simulink model "controllo_Completo_v14"  (R2025a)
settings: Solver=VariableStepAuto  StartTime=0.0  StopTime=Durata_Simulazione  MaxStep=Passo_integrazione_massimo  RelTol=1e-3
values from neighbouring files (symbols this model uses):
  C_bat_eq_rx = 1.0    (= 1)    [p_schema_completo_generale_v2.m]
  C_bat_eq_tx = 3.5    [p_schema_completo_generale_v2.m]
  C_bus_dc_dc = 1.5e-3    (= 0.0015)    [p_schema_completo_generale_v2.m]
  C_ris = 1/(w_dc_ac_nom^2*L_coil)    (= 6.49245057301e-08)    [p_schema_completo_generale_v2.m]
  dead_time_dc_dc = 0.3e-6    (= 3e-07)    [p_schema_completo_generale_v2.m]
  duty_A_0_tx = V_bat_0_tx/V_dc_0_tx    (= 0.472727272727)    [p_schema_completo_generale_v2.m]
  duty_B_0_tx = duty_A_0_tx    (= 0.472727272727)    [p_schema_completo_generale_v2.m]
  duty_leg_A_dc_dc_0_tx = V_bat_0_tx/V_dc_0_tx    (= 0.472727272727)    [p_schema_completo_generale_v2.m]
  duty_leg_B_dc_dc_0_tx = duty_leg_A_dc_dc_0_tx    (= 0.472727272727)    [p_schema_completo_generale_v2.m]
  Ibat_rif_max = 50    [p_schema_completo_generale_v2.m]
  Ibat_rif_min = -50    [p_schema_completo_generale_v2.m]
  Kp_P_tensione_batteria_rx = 1/modulo_catena_aperta_tensione_batteria_reg_P_rx    [p_schema_completo_generale_v2.m]
  Kp_P_tensione_batteria_tx = 1/modulo_catena_aperta_tensione_batteria_reg_P_tx    [p_schema_completo_generale_v2.m]
  L_coil = 54e-6    (= 5.4e-05)    [p_schema_completo_generale_v2.m]
  L_filtro_dc_dc = 65e-6    (= 6.5e-05)    [p_schema_completo_generale_v2.m]
  M_coil = k*sqrt(L_coil^2)    [p_schema_completo_generale_v2.m]
  Parametri_Controllori = [Parametri_Controllori     PI_corrente_trasm_tf_disc_den(2) PI_corrente_trasm_tf_disc_num(1) PI_corrente_trasm_tf_disc_num(2)]    [p_schema_completo_generale_v2.m]
  R_bat = 32e-3    (= 0.032)    [p_schema_completo_generale_v2.m]
  R_coil = w_dc_ac_nom*L_coil/Q_coil    (= 0.2883982056)    [p_schema_completo_generale_v2.m]
  R_coil_M = sqrt(w_dc_ac_nom^2)*M_coil/sqrt(Q_coil^2)    [p_schema_completo_generale_v2.m]
  R_Lfiltro_dc_dc = 6.5e-3    (= 0.0065)    [p_schema_completo_generale_v2.m]
  Req_Lfiltro_dc_dc = (R_Lfiltro_dc_dc+Rds_on_dc_dc)    (= 0.0075)    [p_schema_completo_generale_v2.m]
  Rshunt_coil = 1e5    (= 100000)    [p_schema_completo_generale_v2.m]
  Rshunt_Lfiltro = 1e6    (= 1000000)    [p_schema_completo_generale_v2.m]
  T_dc_ac = 1/freq_dc_ac    (= 1.17647058824e-05)    [p_schema_completo_generale_v2.m]
  T_dc_dc = 1/freq_dc_dc    (= 7.8431372549e-06)    [p_schema_completo_generale_v2.m]
  tau_filtro_anti_aliasing = R_filtro_anti_aliasing*C_filtro_anti_aliasing    (= 1.96e-06)    [p_schema_completo_generale_v2.m]
  tau_filtro_pb_coil = 1/(2*pi*f_filtro_pb_coil)    (= 3.18309886184e-05)    [p_schema_completo_generale_v2.m]
  tau_filtro_pb_corrente_bat = 1/(2*pi*f_filtro_pb_corrente_bat)    (= 2.49654812693e-05)    [p_schema_completo_generale_v2.m]
  Ts_BMS = 1e-3    (= 0.001)    [p_schema_completo_generale_v2.m]
  Ts_dc_ac = 4*T_dc_ac    (= 4.70588235294e-05)    [p_schema_completo_generale_v2.m]
  Ts_dc_dc = Ts_dc_ac    (= 4.70588235294e-05)    [p_schema_completo_generale_v2.m]
  Ts_trasmissione = 1e-3    (= 0.001)    [p_schema_completo_generale_v2.m]
  V_bat_0_rx = V_bat_nom    (= 96)    [p_schema_completo_generale_v2.m]
  V_bat_0_tx = V_bat_max-5    (= 104)    [p_schema_completo_generale_v2.m]
  V_bat_max = 109    [p_schema_completo_generale_v2.m]
  V_bat_max_alg = 218    [Controllo_tensione_bus_dc.m]    (also in Controllo_tensione_bus_dc_corrente_bobina.m; p_schema_completo_generale_v2.m)
  V_bat_min = 75    [p_schema_completo_generale_v2.m]
  V_bat_min_alg = 37.5    [Controllo_tensione_bus_dc.m]    (also in Controllo_tensione_bus_dc_corrente_bobina.m; p_schema_completo_generale_v2.m)
  V_dc_0_rx = 230    [p_schema_completo_generale_v2.m]
  V_dc_0_tx = 220    [p_schema_completo_generale_v2.m]
  Vbat_rif_max_tx = V_bat_max    (= 109)    [p_schema_completo_generale_v2.m]
  Vbat_rif_min_tx = V_bat_min    (= 75)    [p_schema_completo_generale_v2.m]
  Vdc_rif_max_tx = V_dc_nom+5    (= 255)    [p_schema_completo_generale_v2.m]
  Vdc_rif_min_tx = V_dc_nom-5    (= 245)    [p_schema_completo_generale_v2.m]
undefined symbols (not defined in the file or in its folder): Ceq_bat_tx, Cris_tx, Lfilt_dc_dc, Lfiltro_dc_dc_tx, R_bat_rx, R_bat_tx
libraries: simulink x44, spsSeriesRLCBranchLib x36, spsCurrentMeasurementLib x20, spsMosfetLib x16, spsVoltageMeasurementLib x12, simulink_extras x4, spsControlledCurrentSourceLib x4, spsControlledVoltageSourceLib x4, spsDCVoltageSourceLib x2, spsMutualInductanceLib x1, spsGroundLib x1, sps_lib x1
(part 3 of 7)

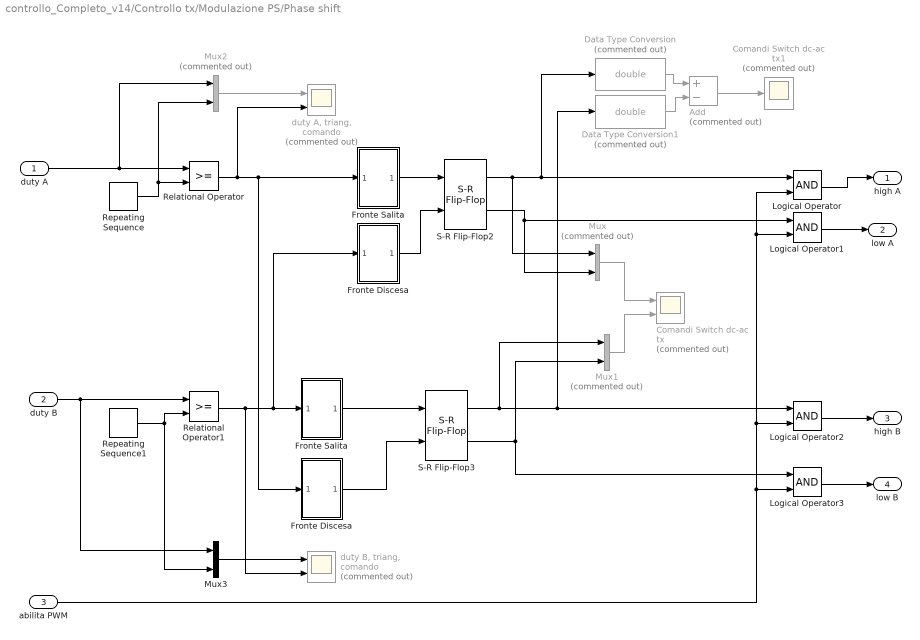
== system controllo_Completo_v14/Controllo tx/Modulazione PS/Phase shift ==
  duty A : Inport
  duty B : Inport  Port=2
  abilita PWM : Inport  Port=3
  Add : Sum  Commented=on  Inputs=+-
  Comandi Switch dc-ac tx : Scope  Commented=on  NumInputPorts=2
      settings: ActiveDisplayYMinimum=-0.12499999999999997  ActiveDisplayYMaximum=1.125  DataLoggingVariableName=ScopeData14
  Comandi Switch dc-ac tx1 : Scope  Commented=on
      settings: ActiveDisplayYMinimum=-1.25  ActiveDisplayYMaximum=1.25  DataLoggingVariableName=ScopeData5
  Data Type Conversion : DataTypeConversion  Commented=on  OutDataTypeStr=double  SaturateOnIntegerOverflow=off  RndMeth=Floor
  Data Type Conversion1 : DataTypeConversion  Commented=on  OutDataTypeStr=double  SaturateOnIntegerOverflow=off  RndMeth=Floor
  Fronte Discesa : Subsystem
  "Fronte Discesa " : Subsystem
  Fronte Salita : Subsystem
  "Fronte Salita " : Subsystem
  Logical Operator{,1..3} (4 alike) : Logic  AllPortsSameDT=off  OutDataTypeStr=boolean
  Mux : Mux  Commented=on  Inputs=2
  Mux1 : Mux  Commented=on  Inputs=2
  Mux2 : Mux  Commented=on  Inputs=2
  Mux3 : Mux  Inputs=2
  Relational Operator : RelationalOperator  OutDataTypeStr=boolean  RndMeth=Simplest  InputSameDT=off
  Relational Operator1 : RelationalOperator  OutDataTypeStr=boolean  RndMeth=Simplest  InputSameDT=off
  Repeating Sequence : simulink/Sources/Repeating Sequence  rep_seq_t=[0 1/2 1]*T_dc_ac  rep_seq_y=[1 0 1]
  Repeating Sequence1 : simulink/Sources/Repeating Sequence  rep_seq_t=[0 1/2 1]*T_dc_ac  rep_seq_y=[1 0 1]
  S-R Flip-Flop2 : simulink_extras/Flip Flops/S-R Flip-Flop  initial_condition=0
  S-R Flip-Flop3 : simulink_extras/Flip Flops/S-R Flip-Flop  initial_condition=0
  "duty A, triang, comando" : Scope  Commented=on  NumInputPorts=2
      settings: ActiveDisplayYMinimum=0.98956207928910589  ActiveDisplayYMaximum=1.00212977441315  DataLoggingVariableName=ScopeData29
  "duty B, triang, comando" : Scope  Commented=on  NumInputPorts=2
      settings: ActiveDisplayYMinimum=-0.12499999999999997  ActiveDisplayYMaximum=1.125  DataLoggingVariableName=ScopeData24
  high A : Outport
  low A : Outport  Port=2
  high B : Outport  Port=3
  low B : Outport  Port=4
  wires:
  Repeating Sequence/1 -> Mux2/2, Relational Operator/2
  duty B/1 -> Mux3/1, Relational Operator1/1
  Relational Operator/1 -> "duty A, triang, comando"/2, "Fronte Discesa "/1(In1), Fronte Salita/1(In1)
  Relational Operator1/1 -> "duty B, triang, comando"/2, "Fronte Salita "/1(In1), Fronte Discesa/1(In1)
  Repeating Sequence1/1 -> Mux3/2, Relational Operator1/2
  duty A/1 -> Mux2/1, Relational Operator/1
  Mux/1 -> Comandi Switch dc-ac tx/1
  Mux1/1 -> Comandi Switch dc-ac tx/2
  Fronte Salita/1(Out1) -> S-R Flip-Flop2/1
  Fronte Discesa/1(Out1) -> S-R Flip-Flop2/2
  S-R Flip-Flop2/1 -> Mux/1, Data Type Conversion/1, Logical Operator/1
  S-R Flip-Flop2/2 -> Mux/2, Logical Operator1/1
  "Fronte Salita "/1(Out1) -> S-R Flip-Flop3/1
  "Fronte Discesa "/1(Out1) -> S-R Flip-Flop3/2
  S-R Flip-Flop3/1 -> Mux1/1, Logical Operator2/1, Data Type Conversion1/1
  S-R Flip-Flop3/2 -> Mux1/2, Logical Operator3/1
  Add/1 -> Comandi Switch dc-ac tx1/1
  Data Type Conversion/1 -> Add/1
  Data Type Conversion1/1 -> Add/2
  Mux2/1 -> "duty A, triang, comando"/1
  Mux3/1 -> "duty B, triang, comando"/1
  Logical Operator/1 -> high A/1
  Logical Operator1/1 -> low A/1
  Logical Operator2/1 -> high B/1
  Logical Operator3/1 -> low B/1
  abilita PWM/1 -> Logical Operator3/2, Logical Operator2/2, Logical Operator1/2, Logical Operator/2

== system controllo_Completo_v14/Controllo tx/Modulazione PWM/Variant Subsystem ==
  high A : Inport
  low A : Inport  Port=2
  high B : Inport  Port=3
  low B : Inport  Port=4
  dead time : Subsystem  VariantControl=(Selettore_No_Dead_Time_0_Dead_Time_1_tx==1)&(Selettore_Switching_0_Valori_Medi_1_dc_dc_tx==0)
  no dead time : Subsystem  VariantControl=(Selettore_No_Dead_Time_0_Dead_Time_1_tx==0)|(Selettore_Switching_0_Valori_Medi_1_dc_dc_tx==1)
  high A DT : Outport
  low A DT : Outport  Port=2
  high B DT : Outport  Port=3
  low B DT : Outport  Port=4

== system controllo_Completo_v14/Controllo tx/Modulazione PWM/Variant Subsystem1 ==
  duty A : Inport
  duty B : Inport  Port=2
  abilita PWM : Inport  Port=3
  Modulazione Lineare : Subsystem  VariantControl=Selettore_Switching_0_Valori_Medi_1_dc_dc_tx==1
  PWM Seno-Triangolo : Subsystem  VariantControl=Selettore_Switching_0_Valori_Medi_1_dc_dc_tx==0
  high A : Outport
  low A : Outport  Port=2
  high B : Outport  Port=3
  low B : Outport  Port=4

== system controllo_Completo_v14/Convertitore dc-dc/Convertitore dc-dc valori medi/Subsystem ==
  From : From  Commented=on  GotoTag=dc_dc_leg_A_high_tx  TagVisibility=global
  From11 : From  Commented=on  GotoTag=v_dc_tx  TagVisibility=global
  From12 : From  Commented=on  GotoTag=v_bat_tx  TagVisibility=global
  From13 : From  Commented=on  GotoTag=v_dc_tx  TagVisibility=global
  From18 : From  Commented=on  GotoTag=v_bat_tx  TagVisibility=global
  From5 : From  Commented=on  GotoTag=dc_dc_leg_B_high_tx  TagVisibility=global
  From7 : From  Commented=on  GotoTag=abilita_PWM_tx  TagVisibility=global
  Product2 : Product  Commented=on
  Product4 : Product  Commented=on
  Switch : Switch  Commented=on  Criteria=u2 > Threshold  Threshold=0.5  SaturateOnIntegerOverflow=off  InputSameDT=off
  Switch1 : Switch  Commented=on  Criteria=u2 > Threshold  Threshold=0.5  SaturateOnIntegerOverflow=off  InputSameDT=off
  Out1 : Outport
  Out2 : Outport  Port=2
  wires:
  From7/1 -> Switch1/2, Switch/2
  From18/1 -> Switch1/3
  From5/1 -> Product4/2
  Product4/1 -> Switch1/1
  From11/1 -> Product2/1
  From12/1 -> Switch/3
  Product2/1 -> Switch/1
  Switch/1 -> Out1/1
  From/1 -> Product2/2
  From13/1 -> Product4/1
  Switch1/1 -> Out2/1

== system controllo_Completo_v14/Convertitore dc-dc /Convertitore dc-dc Valori Medi /Subsystem ==
  From13 : From  Commented=on  GotoTag=dc_dc_leg_A_high_rx  TagVisibility=global
  From14 : From  Commented=on  GotoTag=dc_dc_leg_B_high_rx  TagVisibility=global
  From20 : From  Commented=on  GotoTag=abilita_PWM_rx  TagVisibility=global
  From21 : From  Commented=on  GotoTag=v_dc_rx  TagVisibility=global
  From22 : From  Commented=on  GotoTag=v_bat_rx  TagVisibility=global
  From23 : From  Commented=on  GotoTag=v_dc_rx  TagVisibility=global
  Product3 : Product  Commented=on
  Product8 : Product  Commented=on
  Switch2 : Switch  Commented=on  Criteria=u2 > Threshold  Threshold=0.5  SaturateOnIntegerOverflow=off  InputSameDT=off
  Switch3 : Switch  Commented=on  Criteria=u2 > Threshold  Threshold=0.5  SaturateOnIntegerOverflow=off  InputSameDT=off
  Out1 : Outport
  Out2 : Outport  Port=2
  wires:
  Switch2/1 -> Out1/1
  From14/1 -> Product8/2
  From21/1 -> Product3/1
  Switch3/1 -> Out2/1
  From22/1 -> Switch3/3, Switch2/3
  Product8/1 -> Switch3/1
  Product3/1 -> Switch2/1
  From23/1 -> Product8/1
  From20/1 -> Switch3/2, Switch2/2
  From13/1 -> Product3/2

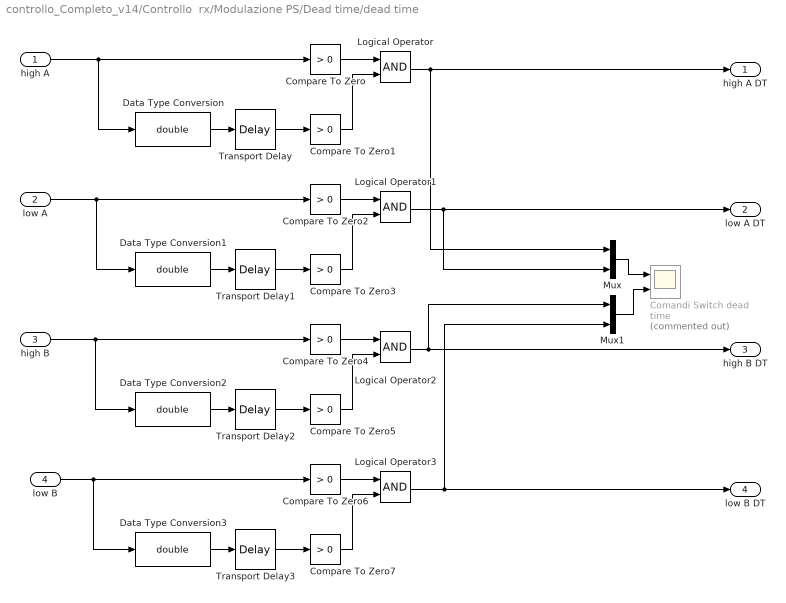
== system controllo_Completo_v14/Controllo  rx/Modulazione PS/Dead time/dead time ==
  high A : Inport
  low A : Inport  Port=2
  high B : Inport  Port=3
  low B : Inport  Port=4
  Comandi Switch dead time : Scope  Commented=on  NumInputPorts=2
      settings: ActiveDisplayYMinimum=-0.12499999999999997  ActiveDisplayYMaximum=1.125  DataLoggingVariableName=ScopeData11
  Compare To Zero{,1..7} (8 alike) : simulink/Logic and Bit Operations/Compare To Zero  relop=>  OutDataTypeStr=boolean
  Data Type Conversion{,1..3} (4 alike) : DataTypeConversion  OutDataTypeStr=double  SaturateOnIntegerOverflow=off  RndMeth=Floor
  Logical Operator{,1..3} (4 alike) : Logic  AllPortsSameDT=off  OutDataTypeStr=boolean
  Mux : Mux  Inputs=2
  Mux1 : Mux  Inputs=2
  Transport Delay{,1..3} (4 alike) : TransportDelay  DelayTime=dead_time_dc_dc
  high A DT : Outport
  low A DT : Outport  Port=2
  high B DT : Outport  Port=3
  low B DT : Outport  Port=4
  wires:
  Mux/1 -> Comandi Switch dead time/1
  Data Type Conversion3/1 -> Transport Delay3/1
  Data Type Conversion2/1 -> Transport Delay2/1
  Data Type Conversion1/1 -> Transport Delay1/1
  Data Type Conversion/1 -> Transport Delay/1
  Mux1/1 -> Comandi Switch dead time/2
  Logical Operator2/1 -> high B DT/1, Mux1/1
  Logical Operator3/1 -> low B DT/1, Mux1/2
  high B/1 -> Data Type Conversion2/1, Compare To Zero4/1
  Transport Delay2/1 -> Compare To Zero5/1
  Compare To Zero5/1 -> Logical Operator2/2
  Compare To Zero4/1 -> Logical Operator2/1
  low B/1 -> Data Type Conversion3/1, Compare To Zero6/1
  Compare To Zero7/1 -> Logical Operator3/2
  Compare To Zero6/1 -> Logical Operator3/1
  Transport Delay3/1 -> Compare To Zero7/1
  Logical Operator1/1 -> low A DT/1, Mux/2
  low A/1 -> Data Type Conversion1/1, Compare To Zero2/1
  Transport Delay1/1 -> Compare To Zero3/1
  Compare To Zero3/1 -> Logical Operator1/2
  Compare To Zero2/1 -> Logical Operator1/1
  Logical Operator/1 -> high A DT/1, Mux/1
  high A/1 -> Data Type Conversion/1, Compare To Zero/1
  Compare To Zero1/1 -> Logical Operator/2
  Transport Delay/1 -> Compare To Zero1/1
  Compare To Zero/1 -> Logical Operator/1

== system controllo_Completo_v14/Controllo  rx/Modulazione PS/Dead time/no dead time ==
  high A : Inport
  low A : Inport  Port=2
  high B : Inport  Port=3
  low B : Inport  Port=4
  high A DT : Outport
  low A DT : Outport  Port=2
  high B DT : Outport  Port=3
  low B DT : Outport  Port=4
  wires:
  low B/1 -> low B DT/1
  high B/1 -> high B DT/1
  low A/1 -> low A DT/1
  high A/1 -> high A DT/1

== system controllo_Completo_v14/Controllo  rx/Modulazione PS/Phase shift/Fronte Discesa ==
  In1 : Inport
  Memory : Memory
  Relational Operator2 : RelationalOperator  Operator=<  OutDataTypeStr=boolean  RndMeth=Simplest  InputSameDT=off
  Out1 : Outport
  wires:
  Relational Operator2/1 -> Out1/1
  In1/1 -> Memory/1, Relational Operator2/1
  Memory/1 -> Relational Operator2/2

== system controllo_Completo_v14/Controllo  rx/Modulazione PS/Phase shift/Fronte Discesa  ==
  In1 : Inport
  Memory : Memory
  Relational Operator2 : RelationalOperator  Operator=<  OutDataTypeStr=boolean  RndMeth=Simplest  InputSameDT=off
  Out1 : Outport
  wires:
  Memory/1 -> Relational Operator2/2
  In1/1 -> Relational Operator2/1, Memory/1
  Relational Operator2/1 -> Out1/1

== system controllo_Completo_v14/Controllo  rx/Modulazione PS/Phase shift/Fronte Salita ==
  In1 : Inport
  Memory : Memory
  Relational Operator2 : RelationalOperator  Operator=>  OutDataTypeStr=boolean  RndMeth=Simplest  InputSameDT=off
  Out1 : Outport
  wires:
  Memory/1 -> Relational Operator2/2
  In1/1 -> Memory/1, Relational Operator2/1
  Relational Operator2/1 -> Out1/1

== system controllo_Completo_v14/Controllo  rx/Modulazione PS/Phase shift/Fronte Salita  ==
  In1 : Inport
  Memory : Memory
  Relational Operator2 : RelationalOperator  Operator=>  OutDataTypeStr=boolean  RndMeth=Simplest  InputSameDT=off
  Out1 : Outport
  wires:
  Relational Operator2/1 -> Out1/1
  In1/1 -> Relational Operator2/1, Memory/1
  Memory/1 -> Relational Operator2/2

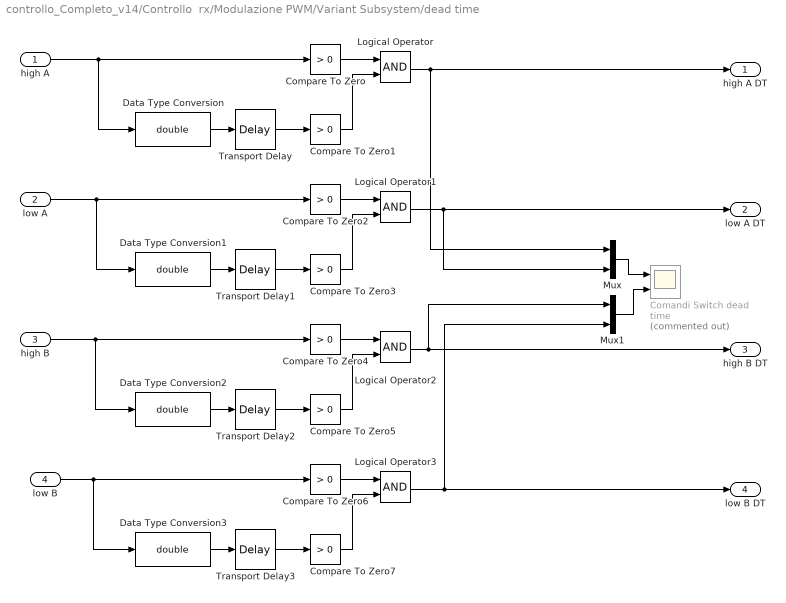
== system controllo_Completo_v14/Controllo  rx/Modulazione PWM/Variant Subsystem/dead time ==
  high A : Inport
  low A : Inport  Port=2
  high B : Inport  Port=3
  low B : Inport  Port=4
  Comandi Switch dead time : Scope  Commented=on  NumInputPorts=2
      settings: ActiveDisplayYMinimum=-0.12499999999999997  ActiveDisplayYMaximum=1.125  DataLoggingVariableName=ScopeData11
  Compare To Zero{,1..7} (8 alike) : simulink/Logic and Bit Operations/Compare To Zero  relop=>  OutDataTypeStr=boolean
  Data Type Conversion{,1..3} (4 alike) : DataTypeConversion  OutDataTypeStr=double  SaturateOnIntegerOverflow=off  RndMeth=Floor
  Logical Operator{,1..3} (4 alike) : Logic  AllPortsSameDT=off  OutDataTypeStr=boolean
  Mux : Mux  Inputs=2
  Mux1 : Mux  Inputs=2
  Transport Delay{,1..3} (4 alike) : TransportDelay  DelayTime=dead_time_dc_dc
  high A DT : Outport
  low A DT : Outport  Port=2
  high B DT : Outport  Port=3
  low B DT : Outport  Port=4
  wires:
  Mux/1 -> Comandi Switch dead time/1
  Data Type Conversion3/1 -> Transport Delay3/1
  Data Type Conversion2/1 -> Transport Delay2/1
  Data Type Conversion1/1 -> Transport Delay1/1
  Data Type Conversion/1 -> Transport Delay/1
  Mux1/1 -> Comandi Switch dead time/2
  Logical Operator2/1 -> high B DT/1, Mux1/1
  Logical Operator3/1 -> low B DT/1, Mux1/2
  high B/1 -> Data Type Conversion2/1, Compare To Zero4/1
  Transport Delay2/1 -> Compare To Zero5/1
  Compare To Zero5/1 -> Logical Operator2/2
  Compare To Zero4/1 -> Logical Operator2/1
  low B/1 -> Data Type Conversion3/1, Compare To Zero6/1
  Compare To Zero7/1 -> Logical Operator3/2
  Compare To Zero6/1 -> Logical Operator3/1
  Transport Delay3/1 -> Compare To Zero7/1
  Logical Operator1/1 -> low A DT/1, Mux/2
  low A/1 -> Data Type Conversion1/1, Compare To Zero2/1
  Transport Delay1/1 -> Compare To Zero3/1
  Compare To Zero3/1 -> Logical Operator1/2
  Compare To Zero2/1 -> Logical Operator1/1
  Logical Operator/1 -> high A DT/1, Mux/1
  high A/1 -> Data Type Conversion/1, Compare To Zero/1
  Compare To Zero1/1 -> Logical Operator/2
  Transport Delay/1 -> Compare To Zero1/1
  Compare To Zero/1 -> Logical Operator/1

== system controllo_Completo_v14/Controllo  rx/Modulazione PWM/Variant Subsystem/no dead time ==
  high A : Inport
  low A : Inport  Port=2
  high B : Inport  Port=3
  low B : Inport  Port=4
  high A DT : Outport
  low A DT : Outport  Port=2
  high B DT : Outport  Port=3
  low B DT : Outport  Port=4
  wires:
  low B/1 -> low B DT/1
  high B/1 -> high B DT/1
  low A/1 -> low A DT/1
  high A/1 -> high A DT/1

== system controllo_Completo_v14/Controllo  rx/Modulazione PWM/Variant Subsystem1/Modulazione Lineare ==
  duty A : Inport
  duty B : Inport  Port=2
  abilita PWM : Inport  Port=3
  Ground : Ground
  Ground1 : Ground
  Terminator : Terminator
  high A : Outport
  low A : Outport  Port=2
  high B : Outport  Port=3
  low B : Outport  Port=4
  wires:
  Ground1/1 -> low B/1
  Ground/1 -> low A/1
  abilita PWM/1 -> Terminator/1
  duty B/1 -> high B/1
  duty A/1 -> high A/1

== system controllo_Completo_v14/Controllo  rx/Modulazione PWM/Variant Subsystem1/PWM Seno-Triangolo ==
  duty A : Inport
  duty B : Inport  Port=2
  abilita PWM : Inport  Port=3
  Logical Operator : Logic  Operator=NOT  AllPortsSameDT=off  OutDataTypeStr=boolean
  Logical Operator1 : Logic  Operator=NOT  AllPortsSameDT=off  OutDataTypeStr=boolean
  Logical Operator{2..5} (4 alike) : Logic  AllPortsSameDT=off  OutDataTypeStr=boolean
  Relational Operator : RelationalOperator  OutDataTypeStr=boolean  RndMeth=Simplest  InputSameDT=off
  Relational Operator1 : RelationalOperator  OutDataTypeStr=boolean  RndMeth=Simplest  InputSameDT=off
  Repeating Sequence : simulink/Sources/Repeating Sequence  rep_seq_t=[0 1/2 1]*T_dc_dc  rep_seq_y=[1 0 1]
  Repeating Sequence1 : simulink/Sources/Repeating Sequence  rep_seq_t=[0 1/2 1]*T_dc_dc  rep_seq_y=[0 1 0]
  "duty A, tri tx" : Scope  Commented=on  NumInputPorts=2
      settings: ActiveDisplayYMinimum=-0.12499999999999148  ActiveDisplayYMaximum=1.1249999999999991  DataLoggingVariableName=ScopeData6
  "duty A, tri tx1" : Scope  Commented=on  NumInputPorts=2
      settings: ActiveDisplayYMinimum=-0.12499999999999997  ActiveDisplayYMaximum=1.125  DataLoggingVariableName=ScopeData12
  "duty A, tri tx2" : Scope  Commented=on  NumInputPorts=2
      settings: ActiveDisplayYMinimum=-0.028634361233479844  ActiveDisplayYMaximum=0.44631057268722485  DataLoggingVariableName=ScopeData13
  high A : Outport
  low A : Outport  Port=2
  high B : Outport  Port=3
  low B : Outport  Port=4
  wires:
  duty B/1 -> Relational Operator1/1
  Relational Operator/1 -> Logical Operator2/2, Logical Operator/1  "block"
  Relational Operator1/1 -> Logical Operator4/2, Logical Operator1/1
  duty A/1 -> "duty A, tri tx2"/2, "duty A, tri tx"/2, Relational Operator/1
  Repeating Sequence/1 -> "duty A, tri tx"/1, Relational Operator/2
  Repeating Sequence1/1 -> Relational Operator1/2
  Logical Operator2/1 -> "duty A, tri tx1"/1, high A/1
  abilita PWM/1 -> "duty A, tri tx2"/1, Logical Operator2/1, Logical Operator3/1, Logical Operator4/1, Logical Operator5/1
  Logical Operator/1 -> Logical Operator3/2
  Logical Operator3/1 -> "duty A, tri tx1"/2, low A/1
  Logical Operator4/1 -> high B/1
  Logical Operator1/1 -> Logical Operator5/2
  Logical Operator5/1 -> low B/1

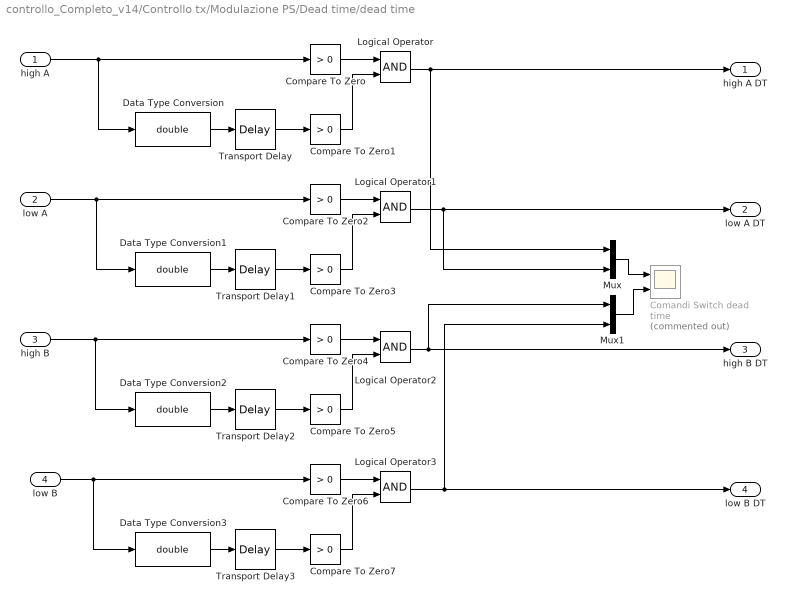
== system controllo_Completo_v14/Controllo tx/Modulazione PS/Dead time/dead time ==
  high A : Inport
  low A : Inport  Port=2
  high B : Inport  Port=3
  low B : Inport  Port=4
  Comandi Switch dead time : Scope  Commented=on  NumInputPorts=2
      settings: ActiveDisplayYMinimum=-0.12499999999999997  ActiveDisplayYMaximum=1.125  DataLoggingVariableName=ScopeData11
  Compare To Zero{,1..7} (8 alike) : simulink/Logic and Bit Operations/Compare To Zero  relop=>  OutDataTypeStr=boolean
  Data Type Conversion{,1..3} (4 alike) : DataTypeConversion  OutDataTypeStr=double  SaturateOnIntegerOverflow=off  RndMeth=Floor
  Logical Operator{,1..3} (4 alike) : Logic  AllPortsSameDT=off  OutDataTypeStr=boolean
  Mux : Mux  Inputs=2
  Mux1 : Mux  Inputs=2
  Transport Delay{,1..3} (4 alike) : TransportDelay  DelayTime=dead_time_dc_dc
  high A DT : Outport
  low A DT : Outport  Port=2
  high B DT : Outport  Port=3
  low B DT : Outport  Port=4
  wires:
  Mux/1 -> Comandi Switch dead time/1
  Data Type Conversion3/1 -> Transport Delay3/1
  Data Type Conversion2/1 -> Transport Delay2/1
  Data Type Conversion1/1 -> Transport Delay1/1
  Data Type Conversion/1 -> Transport Delay/1
  Mux1/1 -> Comandi Switch dead time/2
  Logical Operator2/1 -> high B DT/1, Mux1/1
  Logical Operator3/1 -> low B DT/1, Mux1/2
  high B/1 -> Data Type Conversion2/1, Compare To Zero4/1
  Transport Delay2/1 -> Compare To Zero5/1
  Compare To Zero5/1 -> Logical Operator2/2
  Compare To Zero4/1 -> Logical Operator2/1
  low B/1 -> Data Type Conversion3/1, Compare To Zero6/1
  Compare To Zero7/1 -> Logical Operator3/2
  Compare To Zero6/1 -> Logical Operator3/1
  Transport Delay3/1 -> Compare To Zero7/1
  Logical Operator1/1 -> low A DT/1, Mux/2
  low A/1 -> Data Type Conversion1/1, Compare To Zero2/1
  Transport Delay1/1 -> Compare To Zero3/1
  Compare To Zero3/1 -> Logical Operator1/2
  Compare To Zero2/1 -> Logical Operator1/1
  Logical Operator/1 -> high A DT/1, Mux/1
  high A/1 -> Data Type Conversion/1, Compare To Zero/1
  Compare To Zero1/1 -> Logical Operator/2
  Transport Delay/1 -> Compare To Zero1/1
  Compare To Zero/1 -> Logical Operator/1

== system controllo_Completo_v14/Controllo tx/Modulazione PS/Dead time/no dead time ==
  high A : Inport
  low A : Inport  Port=2
  high B : Inport  Port=3
  low B : Inport  Port=4
  high A DT : Outport
  low A DT : Outport  Port=2
  high B DT : Outport  Port=3
  low B DT : Outport  Port=4
  wires:
  low B/1 -> low B DT/1
  high B/1 -> high B DT/1
  low A/1 -> low A DT/1
  high A/1 -> high A DT/1

== system controllo_Completo_v14/Controllo tx/Modulazione PS/Phase shift/Fronte Discesa ==
  In1 : Inport
  Memory : Memory
  Relational Operator2 : RelationalOperator  Operator=<  OutDataTypeStr=boolean  RndMeth=Simplest  InputSameDT=off
  Out1 : Outport
  wires:
  Relational Operator2/1 -> Out1/1
  In1/1 -> Memory/1, Relational Operator2/1
  Memory/1 -> Relational Operator2/2

== system controllo_Completo_v14/Controllo tx/Modulazione PS/Phase shift/Fronte Discesa  ==
  In1 : Inport
  Memory : Memory
  Relational Operator2 : RelationalOperator  Operator=<  OutDataTypeStr=boolean  RndMeth=Simplest  InputSameDT=off
  Out1 : Outport
  wires:
  Memory/1 -> Relational Operator2/2
  In1/1 -> Relational Operator2/1, Memory/1
  Relational Operator2/1 -> Out1/1

== system controllo_Completo_v14/Controllo tx/Modulazione PS/Phase shift/Fronte Salita ==
  In1 : Inport
  Memory : Memory
  Relational Operator2 : RelationalOperator  Operator=>  OutDataTypeStr=boolean  RndMeth=Simplest  InputSameDT=off
  Out1 : Outport
  wires:
  Memory/1 -> Relational Operator2/2
  In1/1 -> Memory/1, Relational Operator2/1
  Relational Operator2/1 -> Out1/1

== system controllo_Completo_v14/Controllo tx/Modulazione PS/Phase shift/Fronte Salita  ==
  In1 : Inport
  Memory : Memory
  Relational Operator2 : RelationalOperator  Operator=>  OutDataTypeStr=boolean  RndMeth=Simplest  InputSameDT=off
  Out1 : Outport
  wires:
  Relational Operator2/1 -> Out1/1
  In1/1 -> Relational Operator2/1, Memory/1
  Memory/1 -> Relational Operator2/2

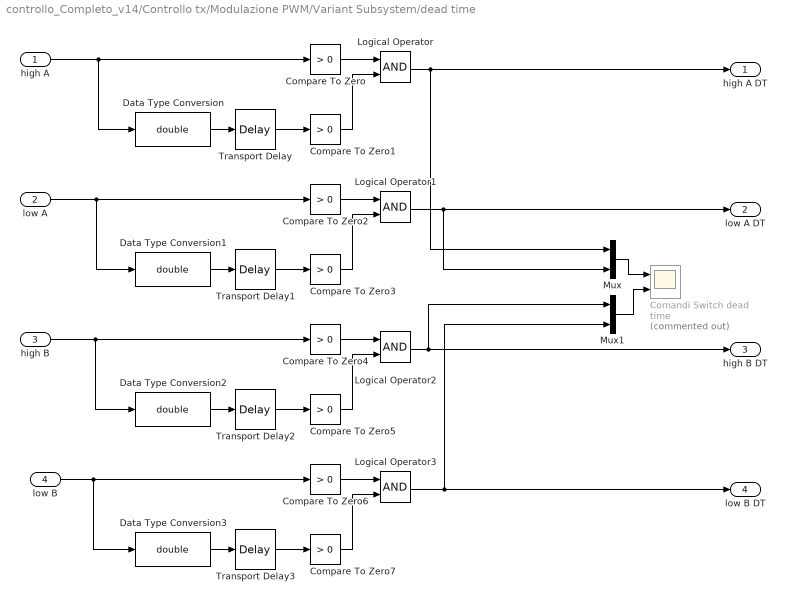
== system controllo_Completo_v14/Controllo tx/Modulazione PWM/Variant Subsystem/dead time ==
  high A : Inport
  low A : Inport  Port=2
  high B : Inport  Port=3
  low B : Inport  Port=4
  Comandi Switch dead time : Scope  Commented=on  NumInputPorts=2
      settings: ActiveDisplayYMinimum=-0.12499999999999997  ActiveDisplayYMaximum=1.125  DataLoggingVariableName=ScopeData11
  Compare To Zero{,1..7} (8 alike) : simulink/Logic and Bit Operations/Compare To Zero  relop=>  OutDataTypeStr=boolean
  Data Type Conversion{,1..3} (4 alike) : DataTypeConversion  OutDataTypeStr=double  SaturateOnIntegerOverflow=off  RndMeth=Floor
  Logical Operator{,1..3} (4 alike) : Logic  AllPortsSameDT=off  OutDataTypeStr=boolean
  Mux : Mux  Inputs=2
  Mux1 : Mux  Inputs=2
  Transport Delay{,1..3} (4 alike) : TransportDelay  DelayTime=dead_time_dc_dc
  high A DT : Outport
  low A DT : Outport  Port=2
  high B DT : Outport  Port=3
  low B DT : Outport  Port=4
  wires:
  Compare To Zero/1 -> Logical Operator/1
  Transport Delay/1 -> Compare To Zero1/1
  Compare To Zero1/1 -> Logical Operator/2
  high A/1 -> Compare To Zero/1, Data Type Conversion/1
  Logical Operator/1 -> Mux/1, high A DT/1
  Compare To Zero2/1 -> Logical Operator1/1
  Compare To Zero3/1 -> Logical Operator1/2
  Transport Delay1/1 -> Compare To Zero3/1
  low A/1 -> Compare To Zero2/1, Data Type Conversion1/1
  Logical Operator1/1 -> Mux/2, low A DT/1
  Transport Delay3/1 -> Compare To Zero7/1
  Compare To Zero6/1 -> Logical Operator3/1
  Compare To Zero7/1 -> Logical Operator3/2
  low B/1 -> Compare To Zero6/1, Data Type Conversion3/1
  Compare To Zero4/1 -> Logical Operator2/1
  Compare To Zero5/1 -> Logical Operator2/2
  Transport Delay2/1 -> Compare To Zero5/1
  high B/1 -> Compare To Zero4/1, Data Type Conversion2/1
  Logical Operator3/1 -> Mux1/2, low B DT/1
  Logical Operator2/1 -> Mux1/1, high B DT/1
  Mux1/1 -> Comandi Switch dead time/2
  Data Type Conversion/1 -> Transport Delay/1
  Data Type Conversion1/1 -> Transport Delay1/1
  Data Type Conversion2/1 -> Transport Delay2/1
  Data Type Conversion3/1 -> Transport Delay3/1
  Mux/1 -> Comandi Switch dead time/1

== system controllo_Completo_v14/Controllo tx/Modulazione PWM/Variant Subsystem/no dead time ==
  high A : Inport
  low A : Inport  Port=2
  high B : Inport  Port=3
  low B : Inport  Port=4
  high A DT : Outport
  low A DT : Outport  Port=2
  high B DT : Outport  Port=3
  low B DT : Outport  Port=4
  wires:
  high A/1 -> high A DT/1
  low A/1 -> low A DT/1
  high B/1 -> high B DT/1
  low B/1 -> low B DT/1

== system controllo_Completo_v14/Controllo tx/Modulazione PWM/Variant Subsystem1/Modulazione Lineare ==
  duty A : Inport
  duty B : Inport  Port=2
  abilita PWM : Inport  Port=3
  Ground : Ground
  Ground1 : Ground
  Terminator : Terminator
  high A : Outport
  low A : Outport  Port=2
  high B : Outport  Port=3
  low B : Outport  Port=4
  wires:
  duty A/1 -> high A/1
  duty B/1 -> high B/1
  abilita PWM/1 -> Terminator/1
  Ground/1 -> low A/1
  Ground1/1 -> low B/1

== system controllo_Completo_v14/Controllo tx/Modulazione PWM/Variant Subsystem1/PWM Seno-Triangolo ==
  duty A : Inport
  duty B : Inport  Port=2
  abilita PWM : Inport  Port=3
  Logical Operator : Logic  Operator=NOT  AllPortsSameDT=off  OutDataTypeStr=boolean
  Logical Operator1 : Logic  Operator=NOT  AllPortsSameDT=off  OutDataTypeStr=boolean
  Logical Operator{2..5} (4 alike) : Logic  AllPortsSameDT=off  OutDataTypeStr=boolean
  Relational Operator : RelationalOperator  OutDataTypeStr=boolean  RndMeth=Simplest  InputSameDT=off
  Relational Operator1 : RelationalOperator  OutDataTypeStr=boolean  RndMeth=Simplest  InputSameDT=off
  Repeating Sequence : simulink/Sources/Repeating Sequence  rep_seq_t=[0 1/2 1]*T_dc_dc  rep_seq_y=[1 0 1]
  Repeating Sequence1 : simulink/Sources/Repeating Sequence  rep_seq_t=[0 1/2 1]*T_dc_dc  rep_seq_y=[0 1 0]
  "duty A, tri tx" : Scope  Commented=on  NumInputPorts=2
      settings: ActiveDisplayYMinimum=-0.12499999999999148  ActiveDisplayYMaximum=1.1249999999999991  DataLoggingDecimation=10  DataLoggingVariableName=ScopeData6
  "duty A, tri tx2" : Scope  Commented=on  NumInputPorts=2
      settings: ActiveDisplayYMinimum=-0.028634361233479844  ActiveDisplayYMaximum=0.44631057268722485  DataLoggingDecimation=10  DataLoggingVariableName=ScopeData13
  "high A, low A, tx" : Scope  Commented=on  NumInputPorts=2
      settings: ActiveDisplayYMinimum=-0.12499999999999997  ActiveDisplayYMaximum=1.125  DataLoggingDecimation=10  DataLoggingVariableName=ScopeData12
  "high B, low B, tx" : Scope  Commented=on  NumInputPorts=2
      settings: ActiveDisplayYMinimum=-0.12499999999999997  ActiveDisplayYMaximum=1.125  DataLoggingDecimation=10  DataLoggingVariableName=ScopeData15
  high A : Outport
  low A : Outport  Port=2
  high B : Outport  Port=3
  low B : Outport  Port=4
  wires:
  Logical Operator5/1 -> "high B, low B, tx"/2, low B/1
  Logical Operator1/1 -> Logical Operator5/2
  Logical Operator4/1 -> "high B, low B, tx"/1, high B/1
  Logical Operator3/1 -> low A/1, "high A, low A, tx"/2
  Logical Operator/1 -> Logical Operator3/2
  abilita PWM/1 -> Logical Operator5/1, Logical Operator4/1, Logical Operator3/1, Logical Operator2/1, "duty A, tri tx2"/1
  Logical Operator2/1 -> high A/1, "high A, low A, tx"/1
  Repeating Sequence1/1 -> Relational Operator1/2
  Repeating Sequence/1 -> Relational Operator/2, "duty A, tri tx"/1
  duty A/1 -> Relational Operator/1, "duty A, tri tx"/2, "duty A, tri tx2"/2
  Relational Operator1/1 -> Logical Operator1/1, Logical Operator4/2
  Relational Operator/1 -> Logical Operator/1, Logical Operator2/2  "block"
  duty B/1 -> Relational Operator1/1

== matlab function controllo_Completo_v14/Convertitore dc-dc /Convertitore dc-dc Valori Medi /MATLAB Function1 ==
  data: Vin output; Abilitazione input; Vdc input; Vbat input; IL input; duty input
function Vin = Simula_dc_dc(Abilitazione, Vdc, Vbat, IL, duty)

    Vin=Vbat;
    
    if(Abilitazione==1)
        Vin=Vdc*duty;
    else
        if(IL>=0.01)
            Vin=Vdc;
        end
        if(IL<=-0.01)
            Vin=0;
        end
        if(abs(IL)<0.01)
            Vin=Vbat;
        end    
    end
